simulink model "TST_PIntkVUs_DD"  (R2016b)
settings: Solver=FixedStepDiscrete  StartTime=0.0  StopTime=simTime  FixedStep=sampleTime  RelTol=1e-3
values from neighbouring files (symbols this model uses):
  testCase = 1    [initTST_PIntkVUs_DD_001.m]    (also in initTST_PIntkVUs_DD_002.m = 2; initTST_PIntkVUs_DD_003.m = 3; initTST_PIntkVUs_DD_004.m = 4; initTST_PIntkVUs_DD_005.m = 5)
libraries: UnitTest_Lib x98, simulink x8
(part 3 of 3)

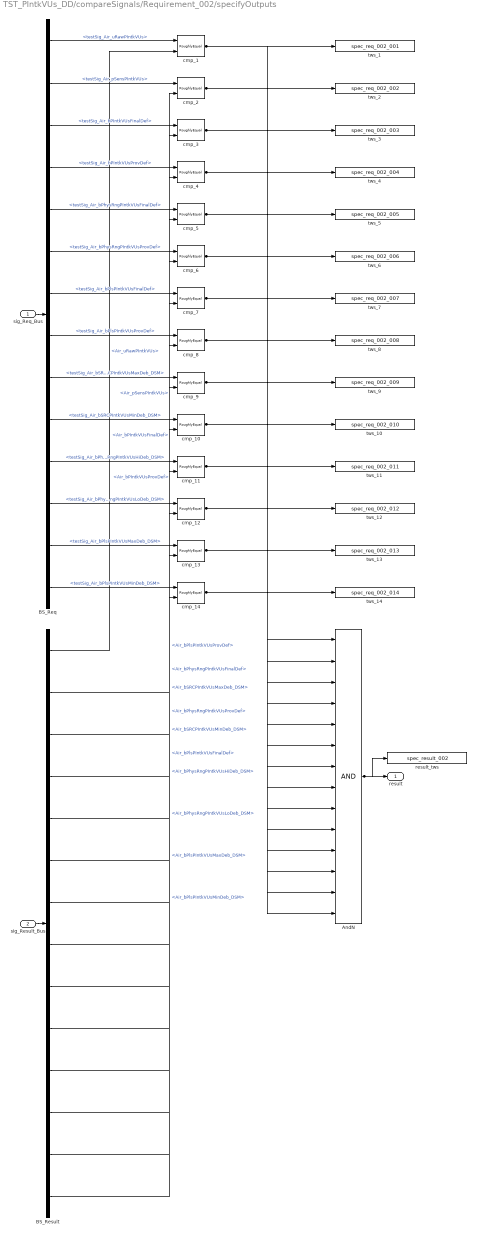
== system TST_PIntkVUs_DD/compareSignals/Requirement_002/specifyOutputs ==
  sig_Req_Bus : Inport
  sig_Result_Bus : Inport  Port=2
  AndN : Logic  Inputs=14
  BS_Req : BusSelector  OutputSignals=testSig_Air_uRawPIntkVUs,testSig_Air_pSensPIntkVUs,testSig_Air_bPIntkVUsFinalDef,testSig_Air_bPIntkVUsProvDef,testSig_Air_bPhysRngPIntkVUsFinalDef,testSig_Air_bPhysRngPIntkVUsProvDef,testSig_Air_bPlsPIntkVUsFinalDef,testSig_Air_bPlsPIntkVUsProvDef,testSig_Air_bSRCPIntkVUsMaxDeb_DSM,testSig_Air_bSRCPIntkVUsMinDeb_DSM,testSig_Air_bPhysRngPIntkVUsHiDeb_DSM,testSig_Air_bPhysRngPIntkVUsLoDeb_DSM,testSig_Air_bPlsPIntkVUsMaxDeb_DSM,testSig_Air_bPlsPIntkVUsMinDeb_DSM
  BS_Result : BusSelector  OutputSignals=Air_uRawPIntkVUs,Air_pSensPIntkVUs,Air_bPIntkVUsFinalDef,Air_bPIntkVUsProvDef,Air_bPhysRngPIntkVUsFinalDef,Air_bPhysRngPIntkVUsProvDef,Air_bPlsPIntkVUsFinalDef,Air_bPlsPIntkVUsProvDef,Air_bSRCPIntkVUsMaxDeb_DSM,Air_bSRCPIntkVUsMinDeb_DSM,Air_bPhysRngPIntkVUsHiDeb_DSM,Air_bPhysRngPIntkVUsLoDeb_DSM,Air_bPlsPIntkVUsMaxDeb_DSM,Air_bPlsPIntkVUsMinDeb_DSM
  cmp_{1..14} (14 alike) : UnitTest_Lib/RoughlyEqual  slope=0.1
  result_tws : ToWorkspace  VariableName=spec_result_002
  tws_1 : ToWorkspace  VariableName=spec_req_002_001
  tws_10 : ToWorkspace  VariableName=spec_req_002_010
  tws_11 : ToWorkspace  VariableName=spec_req_002_011
  tws_12 : ToWorkspace  VariableName=spec_req_002_012
  tws_13 : ToWorkspace  VariableName=spec_req_002_013
  tws_14 : ToWorkspace  VariableName=spec_req_002_014
  tws_2 : ToWorkspace  VariableName=spec_req_002_002
  tws_3 : ToWorkspace  VariableName=spec_req_002_003
  tws_4 : ToWorkspace  VariableName=spec_req_002_004
  tws_5 : ToWorkspace  VariableName=spec_req_002_005
  tws_6 : ToWorkspace  VariableName=spec_req_002_006
  tws_7 : ToWorkspace  VariableName=spec_req_002_007
  tws_8 : ToWorkspace  VariableName=spec_req_002_008
  tws_9 : ToWorkspace  VariableName=spec_req_002_009
  result : Outport
  wires:
  sig_Req_Bus/1 -> BS_Req/1
  sig_Result_Bus/1 -> BS_Result/1
  AndN/1 -> result/1, result_tws/1
  BS_Req/1 -> cmp_1/1  "<testSig_Air_uRawPIntkVUs>"
  BS_Result/1 -> cmp_1/2  "<Air_uRawPIntkVUs>"
  cmp_1/1 -> tws_1/1, AndN/1
  BS_Req/2 -> cmp_2/1  "<testSig_Air_pSensPIntkVUs>"
  BS_Result/2 -> cmp_2/2  "<Air_pSensPIntkVUs>"
  cmp_2/1 -> tws_2/1, AndN/2
  BS_Req/3 -> cmp_3/1  "<testSig_Air_bPIntkVUsFinalDef>"
  BS_Result/3 -> cmp_3/2  "<Air_bPIntkVUsFinalDef>"
  cmp_3/1 -> tws_3/1, AndN/3
  BS_Req/4 -> cmp_4/1  "<testSig_Air_bPIntkVUsProvDef>"
  BS_Result/4 -> cmp_4/2  "<Air_bPIntkVUsProvDef>"
  cmp_4/1 -> tws_4/1, AndN/4
  BS_Req/5 -> cmp_5/1  "<testSig_Air_bPhysRngPIntkVUsFinalDef>"
  BS_Result/5 -> cmp_5/2  "<Air_bPhysRngPIntkVUsFinalDef>"
  cmp_5/1 -> tws_5/1, AndN/5
  BS_Req/6 -> cmp_6/1  "<testSig_Air_bPhysRngPIntkVUsProvDef>"
  BS_Result/6 -> cmp_6/2  "<Air_bPhysRngPIntkVUsProvDef>"
  cmp_6/1 -> tws_6/1, AndN/6
  BS_Req/7 -> cmp_7/1  "<testSig_Air_bPlsPIntkVUsFinalDef>"
  BS_Result/7 -> cmp_7/2  "<Air_bPlsPIntkVUsFinalDef>"
  cmp_7/1 -> tws_7/1, AndN/7
  BS_Req/8 -> cmp_8/1  "<testSig_Air_bPlsPIntkVUsProvDef>"
  BS_Result/8 -> cmp_8/2  "<Air_bPlsPIntkVUsProvDef>"
  cmp_8/1 -> tws_8/1, AndN/8
  BS_Req/9 -> cmp_9/1  "<testSig_Air_bSRCPIntkVUsMaxDeb_DSM>"
  BS_Result/9 -> cmp_9/2  "<Air_bSRCPIntkVUsMaxDeb_DSM>"
  cmp_9/1 -> tws_9/1, AndN/9
  BS_Req/10 -> cmp_10/1  "<testSig_Air_bSRCPIntkVUsMinDeb_DSM>"
  BS_Result/10 -> cmp_10/2  "<Air_bSRCPIntkVUsMinDeb_DSM>"
  cmp_10/1 -> tws_10/1, AndN/10
  BS_Req/11 -> cmp_11/1  "<testSig_Air_bPhysRngPIntkVUsHiDeb_DSM>"
  BS_Result/11 -> cmp_11/2  "<Air_bPhysRngPIntkVUsHiDeb_DSM>"
  cmp_11/1 -> tws_11/1, AndN/11
  BS_Req/12 -> cmp_12/1  "<testSig_Air_bPhysRngPIntkVUsLoDeb_DSM>"
  BS_Result/12 -> cmp_12/2  "<Air_bPhysRngPIntkVUsLoDeb_DSM>"
  cmp_12/1 -> tws_12/1, AndN/12
  BS_Req/13 -> cmp_13/1  "<testSig_Air_bPlsPIntkVUsMaxDeb_DSM>"
  BS_Result/13 -> cmp_13/2  "<Air_bPlsPIntkVUsMaxDeb_DSM>"
  cmp_13/1 -> tws_13/1, AndN/13
  BS_Req/14 -> cmp_14/1  "<testSig_Air_bPlsPIntkVUsMinDeb_DSM>"
  BS_Result/14 -> cmp_14/2  "<Air_bPlsPIntkVUsMinDeb_DSM>"
  cmp_14/1 -> tws_14/1, AndN/14

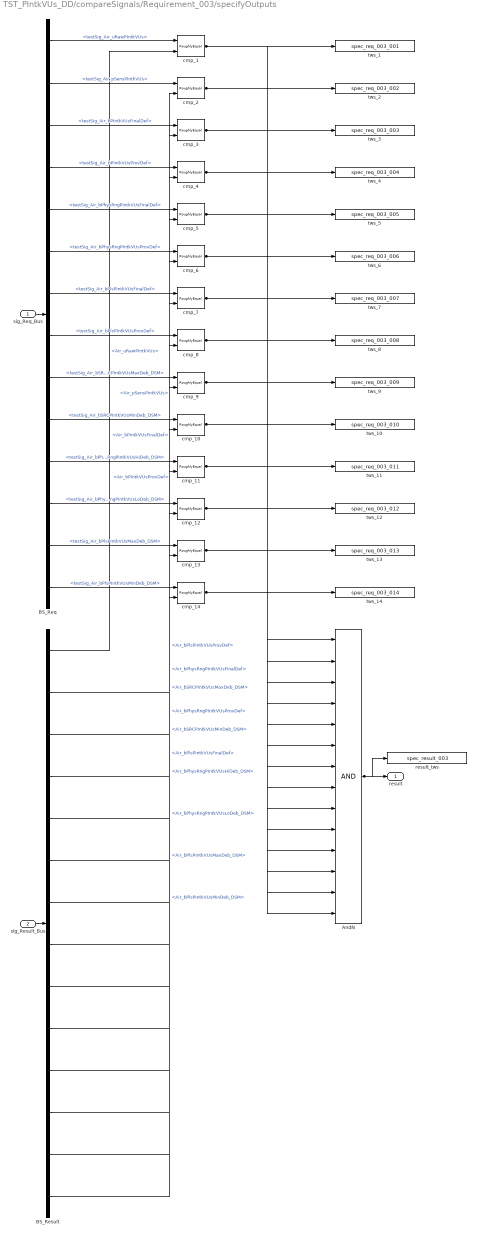
== system TST_PIntkVUs_DD/compareSignals/Requirement_003/specifyOutputs ==
  sig_Req_Bus : Inport
  sig_Result_Bus : Inport  Port=2
  AndN : Logic  Inputs=14
  BS_Req : BusSelector  OutputSignals=testSig_Air_uRawPIntkVUs,testSig_Air_pSensPIntkVUs,testSig_Air_bPIntkVUsFinalDef,testSig_Air_bPIntkVUsProvDef,testSig_Air_bPhysRngPIntkVUsFinalDef,testSig_Air_bPhysRngPIntkVUsProvDef,testSig_Air_bPlsPIntkVUsFinalDef,testSig_Air_bPlsPIntkVUsProvDef,testSig_Air_bSRCPIntkVUsMaxDeb_DSM,testSig_Air_bSRCPIntkVUsMinDeb_DSM,testSig_Air_bPhysRngPIntkVUsHiDeb_DSM,testSig_Air_bPhysRngPIntkVUsLoDeb_DSM,testSig_Air_bPlsPIntkVUsMaxDeb_DSM,testSig_Air_bPlsPIntkVUsMinDeb_DSM
  BS_Result : BusSelector  OutputSignals=Air_uRawPIntkVUs,Air_pSensPIntkVUs,Air_bPIntkVUsFinalDef,Air_bPIntkVUsProvDef,Air_bPhysRngPIntkVUsFinalDef,Air_bPhysRngPIntkVUsProvDef,Air_bPlsPIntkVUsFinalDef,Air_bPlsPIntkVUsProvDef,Air_bSRCPIntkVUsMaxDeb_DSM,Air_bSRCPIntkVUsMinDeb_DSM,Air_bPhysRngPIntkVUsHiDeb_DSM,Air_bPhysRngPIntkVUsLoDeb_DSM,Air_bPlsPIntkVUsMaxDeb_DSM,Air_bPlsPIntkVUsMinDeb_DSM
  cmp_{1..14} (14 alike) : UnitTest_Lib/RoughlyEqual  slope=0.1
  result_tws : ToWorkspace  VariableName=spec_result_003
  tws_1 : ToWorkspace  VariableName=spec_req_003_001
  tws_10 : ToWorkspace  VariableName=spec_req_003_010
  tws_11 : ToWorkspace  VariableName=spec_req_003_011
  tws_12 : ToWorkspace  VariableName=spec_req_003_012
  tws_13 : ToWorkspace  VariableName=spec_req_003_013
  tws_14 : ToWorkspace  VariableName=spec_req_003_014
  tws_2 : ToWorkspace  VariableName=spec_req_003_002
  tws_3 : ToWorkspace  VariableName=spec_req_003_003
  tws_4 : ToWorkspace  VariableName=spec_req_003_004
  tws_5 : ToWorkspace  VariableName=spec_req_003_005
  tws_6 : ToWorkspace  VariableName=spec_req_003_006
  tws_7 : ToWorkspace  VariableName=spec_req_003_007
  tws_8 : ToWorkspace  VariableName=spec_req_003_008
  tws_9 : ToWorkspace  VariableName=spec_req_003_009
  result : Outport
  wires:
  sig_Req_Bus/1 -> BS_Req/1
  sig_Result_Bus/1 -> BS_Result/1
  AndN/1 -> result/1, result_tws/1
  BS_Req/1 -> cmp_1/1  "<testSig_Air_uRawPIntkVUs>"
  BS_Result/1 -> cmp_1/2  "<Air_uRawPIntkVUs>"
  cmp_1/1 -> tws_1/1, AndN/1
  BS_Req/2 -> cmp_2/1  "<testSig_Air_pSensPIntkVUs>"
  BS_Result/2 -> cmp_2/2  "<Air_pSensPIntkVUs>"
  cmp_2/1 -> tws_2/1, AndN/2
  BS_Req/3 -> cmp_3/1  "<testSig_Air_bPIntkVUsFinalDef>"
  BS_Result/3 -> cmp_3/2  "<Air_bPIntkVUsFinalDef>"
  cmp_3/1 -> tws_3/1, AndN/3
  BS_Req/4 -> cmp_4/1  "<testSig_Air_bPIntkVUsProvDef>"
  BS_Result/4 -> cmp_4/2  "<Air_bPIntkVUsProvDef>"
  cmp_4/1 -> tws_4/1, AndN/4
  BS_Req/5 -> cmp_5/1  "<testSig_Air_bPhysRngPIntkVUsFinalDef>"
  BS_Result/5 -> cmp_5/2  "<Air_bPhysRngPIntkVUsFinalDef>"
  cmp_5/1 -> tws_5/1, AndN/5
  BS_Req/6 -> cmp_6/1  "<testSig_Air_bPhysRngPIntkVUsProvDef>"
  BS_Result/6 -> cmp_6/2  "<Air_bPhysRngPIntkVUsProvDef>"
  cmp_6/1 -> tws_6/1, AndN/6
  BS_Req/7 -> cmp_7/1  "<testSig_Air_bPlsPIntkVUsFinalDef>"
  BS_Result/7 -> cmp_7/2  "<Air_bPlsPIntkVUsFinalDef>"
  cmp_7/1 -> tws_7/1, AndN/7
  BS_Req/8 -> cmp_8/1  "<testSig_Air_bPlsPIntkVUsProvDef>"
  BS_Result/8 -> cmp_8/2  "<Air_bPlsPIntkVUsProvDef>"
  cmp_8/1 -> tws_8/1, AndN/8
  BS_Req/9 -> cmp_9/1  "<testSig_Air_bSRCPIntkVUsMaxDeb_DSM>"
  BS_Result/9 -> cmp_9/2  "<Air_bSRCPIntkVUsMaxDeb_DSM>"
  cmp_9/1 -> tws_9/1, AndN/9
  BS_Req/10 -> cmp_10/1  "<testSig_Air_bSRCPIntkVUsMinDeb_DSM>"
  BS_Result/10 -> cmp_10/2  "<Air_bSRCPIntkVUsMinDeb_DSM>"
  cmp_10/1 -> tws_10/1, AndN/10
  BS_Req/11 -> cmp_11/1  "<testSig_Air_bPhysRngPIntkVUsHiDeb_DSM>"
  BS_Result/11 -> cmp_11/2  "<Air_bPhysRngPIntkVUsHiDeb_DSM>"
  cmp_11/1 -> tws_11/1, AndN/11
  BS_Req/12 -> cmp_12/1  "<testSig_Air_bPhysRngPIntkVUsLoDeb_DSM>"
  BS_Result/12 -> cmp_12/2  "<Air_bPhysRngPIntkVUsLoDeb_DSM>"
  cmp_12/1 -> tws_12/1, AndN/12
  BS_Req/13 -> cmp_13/1  "<testSig_Air_bPlsPIntkVUsMaxDeb_DSM>"
  BS_Result/13 -> cmp_13/2  "<Air_bPlsPIntkVUsMaxDeb_DSM>"
  cmp_13/1 -> tws_13/1, AndN/13
  BS_Req/14 -> cmp_14/1  "<testSig_Air_bPlsPIntkVUsMinDeb_DSM>"
  BS_Result/14 -> cmp_14/2  "<Air_bPlsPIntkVUsMinDeb_DSM>"
  cmp_14/1 -> tws_14/1, AndN/14

== system TST_PIntkVUs_DD/compareSignals/Requirement_004/specifyOutputs ==
  sig_Req_Bus : Inport
  sig_Result_Bus : Inport  Port=2
  AndN : Logic  Inputs=14
  BS_Req : BusSelector  OutputSignals=testSig_Air_uRawPIntkVUs,testSig_Air_pSensPIntkVUs,testSig_Air_bPIntkVUsFinalDef,testSig_Air_bPIntkVUsProvDef,testSig_Air_bPhysRngPIntkVUsFinalDef,testSig_Air_bPhysRngPIntkVUsProvDef,testSig_Air_bPlsPIntkVUsFinalDef,testSig_Air_bPlsPIntkVUsProvDef,testSig_Air_bSRCPIntkVUsMaxDeb_DSM,testSig_Air_bSRCPIntkVUsMinDeb_DSM,testSig_Air_bPhysRngPIntkVUsHiDeb_DSM,testSig_Air_bPhysRngPIntkVUsLoDeb_DSM,testSig_Air_bPlsPIntkVUsMaxDeb_DSM,testSig_Air_bPlsPIntkVUsMinDeb_DSM
  BS_Result : BusSelector  OutputSignals=Air_uRawPIntkVUs,Air_pSensPIntkVUs,Air_bPIntkVUsFinalDef,Air_bPIntkVUsProvDef,Air_bPhysRngPIntkVUsFinalDef,Air_bPhysRngPIntkVUsProvDef,Air_bPlsPIntkVUsFinalDef,Air_bPlsPIntkVUsProvDef,Air_bSRCPIntkVUsMaxDeb_DSM,Air_bSRCPIntkVUsMinDeb_DSM,Air_bPhysRngPIntkVUsHiDeb_DSM,Air_bPhysRngPIntkVUsLoDeb_DSM,Air_bPlsPIntkVUsMaxDeb_DSM,Air_bPlsPIntkVUsMinDeb_DSM
  cmp_{1..14} (14 alike) : UnitTest_Lib/RoughlyEqual  slope=0.1
  result_tws : ToWorkspace  VariableName=spec_result_004
  tws_1 : ToWorkspace  VariableName=spec_req_004_001
  tws_10 : ToWorkspace  VariableName=spec_req_004_010
  tws_11 : ToWorkspace  VariableName=spec_req_004_011
  tws_12 : ToWorkspace  VariableName=spec_req_004_012
  tws_13 : ToWorkspace  VariableName=spec_req_004_013
  tws_14 : ToWorkspace  VariableName=spec_req_004_014
  tws_2 : ToWorkspace  VariableName=spec_req_004_002
  tws_3 : ToWorkspace  VariableName=spec_req_004_003
  tws_4 : ToWorkspace  VariableName=spec_req_004_004
  tws_5 : ToWorkspace  VariableName=spec_req_004_005
  tws_6 : ToWorkspace  VariableName=spec_req_004_006
  tws_7 : ToWorkspace  VariableName=spec_req_004_007
  tws_8 : ToWorkspace  VariableName=spec_req_004_008
  tws_9 : ToWorkspace  VariableName=spec_req_004_009
  result : Outport
  wires:
  sig_Req_Bus/1 -> BS_Req/1
  sig_Result_Bus/1 -> BS_Result/1
  AndN/1 -> result/1, result_tws/1
  BS_Req/1 -> cmp_1/1  "<testSig_Air_uRawPIntkVUs>"
  BS_Result/1 -> cmp_1/2  "<Air_uRawPIntkVUs>"
  cmp_1/1 -> tws_1/1, AndN/1
  BS_Req/2 -> cmp_2/1  "<testSig_Air_pSensPIntkVUs>"
  BS_Result/2 -> cmp_2/2  "<Air_pSensPIntkVUs>"
  cmp_2/1 -> tws_2/1, AndN/2
  BS_Req/3 -> cmp_3/1  "<testSig_Air_bPIntkVUsFinalDef>"
  BS_Result/3 -> cmp_3/2  "<Air_bPIntkVUsFinalDef>"
  cmp_3/1 -> tws_3/1, AndN/3
  BS_Req/4 -> cmp_4/1  "<testSig_Air_bPIntkVUsProvDef>"
  BS_Result/4 -> cmp_4/2  "<Air_bPIntkVUsProvDef>"
  cmp_4/1 -> tws_4/1, AndN/4
  BS_Req/5 -> cmp_5/1  "<testSig_Air_bPhysRngPIntkVUsFinalDef>"
  BS_Result/5 -> cmp_5/2  "<Air_bPhysRngPIntkVUsFinalDef>"
  cmp_5/1 -> tws_5/1, AndN/5
  BS_Req/6 -> cmp_6/1  "<testSig_Air_bPhysRngPIntkVUsProvDef>"
  BS_Result/6 -> cmp_6/2  "<Air_bPhysRngPIntkVUsProvDef>"
  cmp_6/1 -> tws_6/1, AndN/6
  BS_Req/7 -> cmp_7/1  "<testSig_Air_bPlsPIntkVUsFinalDef>"
  BS_Result/7 -> cmp_7/2  "<Air_bPlsPIntkVUsFinalDef>"
  cmp_7/1 -> tws_7/1, AndN/7
  BS_Req/8 -> cmp_8/1  "<testSig_Air_bPlsPIntkVUsProvDef>"
  BS_Result/8 -> cmp_8/2  "<Air_bPlsPIntkVUsProvDef>"
  cmp_8/1 -> tws_8/1, AndN/8
  BS_Req/9 -> cmp_9/1  "<testSig_Air_bSRCPIntkVUsMaxDeb_DSM>"
  BS_Result/9 -> cmp_9/2  "<Air_bSRCPIntkVUsMaxDeb_DSM>"
  cmp_9/1 -> tws_9/1, AndN/9
  BS_Req/10 -> cmp_10/1  "<testSig_Air_bSRCPIntkVUsMinDeb_DSM>"
  BS_Result/10 -> cmp_10/2  "<Air_bSRCPIntkVUsMinDeb_DSM>"
  cmp_10/1 -> tws_10/1, AndN/10
  BS_Req/11 -> cmp_11/1  "<testSig_Air_bPhysRngPIntkVUsHiDeb_DSM>"
  BS_Result/11 -> cmp_11/2  "<Air_bPhysRngPIntkVUsHiDeb_DSM>"
  cmp_11/1 -> tws_11/1, AndN/11
  BS_Req/12 -> cmp_12/1  "<testSig_Air_bPhysRngPIntkVUsLoDeb_DSM>"
  BS_Result/12 -> cmp_12/2  "<Air_bPhysRngPIntkVUsLoDeb_DSM>"
  cmp_12/1 -> tws_12/1, AndN/12
  BS_Req/13 -> cmp_13/1  "<testSig_Air_bPlsPIntkVUsMaxDeb_DSM>"
  BS_Result/13 -> cmp_13/2  "<Air_bPlsPIntkVUsMaxDeb_DSM>"
  cmp_13/1 -> tws_13/1, AndN/13
  BS_Req/14 -> cmp_14/1  "<testSig_Air_bPlsPIntkVUsMinDeb_DSM>"
  BS_Result/14 -> cmp_14/2  "<Air_bPlsPIntkVUsMinDeb_DSM>"
  cmp_14/1 -> tws_14/1, AndN/14

== system TST_PIntkVUs_DD/compareSignals/Requirement_005/specifyOutputs ==
  sig_Req_Bus : Inport
  sig_Result_Bus : Inport  Port=2
  AndN : Logic  Inputs=14
  BS_Req : BusSelector  OutputSignals=testSig_Air_uRawPIntkVUs,testSig_Air_pSensPIntkVUs,testSig_Air_bPIntkVUsFinalDef,testSig_Air_bPIntkVUsProvDef,testSig_Air_bPhysRngPIntkVUsFinalDef,testSig_Air_bPhysRngPIntkVUsProvDef,testSig_Air_bPlsPIntkVUsFinalDef,testSig_Air_bPlsPIntkVUsProvDef,testSig_Air_bSRCPIntkVUsMaxDeb_DSM,testSig_Air_bSRCPIntkVUsMinDeb_DSM,testSig_Air_bPhysRngPIntkVUsHiDeb_DSM,testSig_Air_bPhysRngPIntkVUsLoDeb_DSM,testSig_Air_bPlsPIntkVUsMaxDeb_DSM,testSig_Air_bPlsPIntkVUsMinDeb_DSM
  BS_Result : BusSelector  OutputSignals=Air_uRawPIntkVUs,Air_pSensPIntkVUs,Air_bPIntkVUsFinalDef,Air_bPIntkVUsProvDef,Air_bPhysRngPIntkVUsFinalDef,Air_bPhysRngPIntkVUsProvDef,Air_bPlsPIntkVUsFinalDef,Air_bPlsPIntkVUsProvDef,Air_bSRCPIntkVUsMaxDeb_DSM,Air_bSRCPIntkVUsMinDeb_DSM,Air_bPhysRngPIntkVUsHiDeb_DSM,Air_bPhysRngPIntkVUsLoDeb_DSM,Air_bPlsPIntkVUsMaxDeb_DSM,Air_bPlsPIntkVUsMinDeb_DSM
  cmp_{1..14} (14 alike) : UnitTest_Lib/RoughlyEqual  slope=0.1
  result_tws : ToWorkspace  VariableName=spec_result_005
  tws_1 : ToWorkspace  VariableName=spec_req_005_001
  tws_10 : ToWorkspace  VariableName=spec_req_005_010
  tws_11 : ToWorkspace  VariableName=spec_req_005_011
  tws_12 : ToWorkspace  VariableName=spec_req_005_012
  tws_13 : ToWorkspace  VariableName=spec_req_005_013
  tws_14 : ToWorkspace  VariableName=spec_req_005_014
  tws_2 : ToWorkspace  VariableName=spec_req_005_002
  tws_3 : ToWorkspace  VariableName=spec_req_005_003
  tws_4 : ToWorkspace  VariableName=spec_req_005_004
  tws_5 : ToWorkspace  VariableName=spec_req_005_005
  tws_6 : ToWorkspace  VariableName=spec_req_005_006
  tws_7 : ToWorkspace  VariableName=spec_req_005_007
  tws_8 : ToWorkspace  VariableName=spec_req_005_008
  tws_9 : ToWorkspace  VariableName=spec_req_005_009
  result : Outport
  wires:
  sig_Req_Bus/1 -> BS_Req/1
  sig_Result_Bus/1 -> BS_Result/1
  AndN/1 -> result/1, result_tws/1
  BS_Req/1 -> cmp_1/1  "<testSig_Air_uRawPIntkVUs>"
  BS_Result/1 -> cmp_1/2  "<Air_uRawPIntkVUs>"
  cmp_1/1 -> tws_1/1, AndN/1
  BS_Req/2 -> cmp_2/1  "<testSig_Air_pSensPIntkVUs>"
  BS_Result/2 -> cmp_2/2  "<Air_pSensPIntkVUs>"
  cmp_2/1 -> tws_2/1, AndN/2
  BS_Req/3 -> cmp_3/1  "<testSig_Air_bPIntkVUsFinalDef>"
  BS_Result/3 -> cmp_3/2  "<Air_bPIntkVUsFinalDef>"
  cmp_3/1 -> tws_3/1, AndN/3
  BS_Req/4 -> cmp_4/1  "<testSig_Air_bPIntkVUsProvDef>"
  BS_Result/4 -> cmp_4/2  "<Air_bPIntkVUsProvDef>"
  cmp_4/1 -> tws_4/1, AndN/4
  BS_Req/5 -> cmp_5/1  "<testSig_Air_bPhysRngPIntkVUsFinalDef>"
  BS_Result/5 -> cmp_5/2  "<Air_bPhysRngPIntkVUsFinalDef>"
  cmp_5/1 -> tws_5/1, AndN/5
  BS_Req/6 -> cmp_6/1  "<testSig_Air_bPhysRngPIntkVUsProvDef>"
  BS_Result/6 -> cmp_6/2  "<Air_bPhysRngPIntkVUsProvDef>"
  cmp_6/1 -> tws_6/1, AndN/6
  BS_Req/7 -> cmp_7/1  "<testSig_Air_bPlsPIntkVUsFinalDef>"
  BS_Result/7 -> cmp_7/2  "<Air_bPlsPIntkVUsFinalDef>"
  cmp_7/1 -> tws_7/1, AndN/7
  BS_Req/8 -> cmp_8/1  "<testSig_Air_bPlsPIntkVUsProvDef>"
  BS_Result/8 -> cmp_8/2  "<Air_bPlsPIntkVUsProvDef>"
  cmp_8/1 -> tws_8/1, AndN/8
  BS_Req/9 -> cmp_9/1  "<testSig_Air_bSRCPIntkVUsMaxDeb_DSM>"
  BS_Result/9 -> cmp_9/2  "<Air_bSRCPIntkVUsMaxDeb_DSM>"
  cmp_9/1 -> tws_9/1, AndN/9
  BS_Req/10 -> cmp_10/1  "<testSig_Air_bSRCPIntkVUsMinDeb_DSM>"
  BS_Result/10 -> cmp_10/2  "<Air_bSRCPIntkVUsMinDeb_DSM>"
  cmp_10/1 -> tws_10/1, AndN/10
  BS_Req/11 -> cmp_11/1  "<testSig_Air_bPhysRngPIntkVUsHiDeb_DSM>"
  BS_Result/11 -> cmp_11/2  "<Air_bPhysRngPIntkVUsHiDeb_DSM>"
  cmp_11/1 -> tws_11/1, AndN/11
  BS_Req/12 -> cmp_12/1  "<testSig_Air_bPhysRngPIntkVUsLoDeb_DSM>"
  BS_Result/12 -> cmp_12/2  "<Air_bPhysRngPIntkVUsLoDeb_DSM>"
  cmp_12/1 -> tws_12/1, AndN/12
  BS_Req/13 -> cmp_13/1  "<testSig_Air_bPlsPIntkVUsMaxDeb_DSM>"
  BS_Result/13 -> cmp_13/2  "<Air_bPlsPIntkVUsMaxDeb_DSM>"
  cmp_13/1 -> tws_13/1, AndN/13
  BS_Req/14 -> cmp_14/1  "<testSig_Air_bPlsPIntkVUsMinDeb_DSM>"
  BS_Result/14 -> cmp_14/2  "<Air_bPlsPIntkVUsMinDeb_DSM>"
  cmp_14/1 -> tws_14/1, AndN/14

== system TST_PIntkVUs_DD/compareSignals/Requirement_006/specifyOutputs ==
  sig_Req_Bus : Inport
  sig_Result_Bus : Inport  Port=2
  AndN : Logic  Inputs=14
  BS_Req : BusSelector  OutputSignals=testSig_Air_uRawPIntkVUs,testSig_Air_pSensPIntkVUs,testSig_Air_bPIntkVUsFinalDef,testSig_Air_bPIntkVUsProvDef,testSig_Air_bPhysRngPIntkVUsFinalDef,testSig_Air_bPhysRngPIntkVUsProvDef,testSig_Air_bPlsPIntkVUsFinalDef,testSig_Air_bPlsPIntkVUsProvDef,testSig_Air_bSRCPIntkVUsMaxDeb_DSM,testSig_Air_bSRCPIntkVUsMinDeb_DSM,testSig_Air_bPhysRngPIntkVUsHiDeb_DSM,testSig_Air_bPhysRngPIntkVUsLoDeb_DSM,testSig_Air_bPlsPIntkVUsMaxDeb_DSM,testSig_Air_bPlsPIntkVUsMinDeb_DSM
  BS_Result : BusSelector  OutputSignals=Air_uRawPIntkVUs,Air_pSensPIntkVUs,Air_bPIntkVUsFinalDef,Air_bPIntkVUsProvDef,Air_bPhysRngPIntkVUsFinalDef,Air_bPhysRngPIntkVUsProvDef,Air_bPlsPIntkVUsFinalDef,Air_bPlsPIntkVUsProvDef,Air_bSRCPIntkVUsMaxDeb_DSM,Air_bSRCPIntkVUsMinDeb_DSM,Air_bPhysRngPIntkVUsHiDeb_DSM,Air_bPhysRngPIntkVUsLoDeb_DSM,Air_bPlsPIntkVUsMaxDeb_DSM,Air_bPlsPIntkVUsMinDeb_DSM
  cmp_{1..14} (14 alike) : UnitTest_Lib/RoughlyEqual  slope=0.1
  result_tws : ToWorkspace  VariableName=spec_result_006
  tws_1 : ToWorkspace  VariableName=spec_req_006_001
  tws_10 : ToWorkspace  VariableName=spec_req_006_010
  tws_11 : ToWorkspace  VariableName=spec_req_006_011
  tws_12 : ToWorkspace  VariableName=spec_req_006_012
  tws_13 : ToWorkspace  VariableName=spec_req_006_013
  tws_14 : ToWorkspace  VariableName=spec_req_006_014
  tws_2 : ToWorkspace  VariableName=spec_req_006_002
  tws_3 : ToWorkspace  VariableName=spec_req_006_003
  tws_4 : ToWorkspace  VariableName=spec_req_006_004
  tws_5 : ToWorkspace  VariableName=spec_req_006_005
  tws_6 : ToWorkspace  VariableName=spec_req_006_006
  tws_7 : ToWorkspace  VariableName=spec_req_006_007
  tws_8 : ToWorkspace  VariableName=spec_req_006_008
  tws_9 : ToWorkspace  VariableName=spec_req_006_009
  result : Outport
  wires:
  sig_Req_Bus/1 -> BS_Req/1
  sig_Result_Bus/1 -> BS_Result/1
  AndN/1 -> result/1, result_tws/1
  BS_Req/1 -> cmp_1/1  "<testSig_Air_uRawPIntkVUs>"
  BS_Result/1 -> cmp_1/2  "<Air_uRawPIntkVUs>"
  cmp_1/1 -> tws_1/1, AndN/1
  BS_Req/2 -> cmp_2/1  "<testSig_Air_pSensPIntkVUs>"
  BS_Result/2 -> cmp_2/2  "<Air_pSensPIntkVUs>"
  cmp_2/1 -> tws_2/1, AndN/2
  BS_Req/3 -> cmp_3/1  "<testSig_Air_bPIntkVUsFinalDef>"
  BS_Result/3 -> cmp_3/2  "<Air_bPIntkVUsFinalDef>"
  cmp_3/1 -> tws_3/1, AndN/3
  BS_Req/4 -> cmp_4/1  "<testSig_Air_bPIntkVUsProvDef>"
  BS_Result/4 -> cmp_4/2  "<Air_bPIntkVUsProvDef>"
  cmp_4/1 -> tws_4/1, AndN/4
  BS_Req/5 -> cmp_5/1  "<testSig_Air_bPhysRngPIntkVUsFinalDef>"
  BS_Result/5 -> cmp_5/2  "<Air_bPhysRngPIntkVUsFinalDef>"
  cmp_5/1 -> tws_5/1, AndN/5
  BS_Req/6 -> cmp_6/1  "<testSig_Air_bPhysRngPIntkVUsProvDef>"
  BS_Result/6 -> cmp_6/2  "<Air_bPhysRngPIntkVUsProvDef>"
  cmp_6/1 -> tws_6/1, AndN/6
  BS_Req/7 -> cmp_7/1  "<testSig_Air_bPlsPIntkVUsFinalDef>"
  BS_Result/7 -> cmp_7/2  "<Air_bPlsPIntkVUsFinalDef>"
  cmp_7/1 -> tws_7/1, AndN/7
  BS_Req/8 -> cmp_8/1  "<testSig_Air_bPlsPIntkVUsProvDef>"
  BS_Result/8 -> cmp_8/2  "<Air_bPlsPIntkVUsProvDef>"
  cmp_8/1 -> tws_8/1, AndN/8
  BS_Req/9 -> cmp_9/1  "<testSig_Air_bSRCPIntkVUsMaxDeb_DSM>"
  BS_Result/9 -> cmp_9/2  "<Air_bSRCPIntkVUsMaxDeb_DSM>"
  cmp_9/1 -> tws_9/1, AndN/9
  BS_Req/10 -> cmp_10/1  "<testSig_Air_bSRCPIntkVUsMinDeb_DSM>"
  BS_Result/10 -> cmp_10/2  "<Air_bSRCPIntkVUsMinDeb_DSM>"
  cmp_10/1 -> tws_10/1, AndN/10
  BS_Req/11 -> cmp_11/1  "<testSig_Air_bPhysRngPIntkVUsHiDeb_DSM>"
  BS_Result/11 -> cmp_11/2  "<Air_bPhysRngPIntkVUsHiDeb_DSM>"
  cmp_11/1 -> tws_11/1, AndN/11
  BS_Req/12 -> cmp_12/1  "<testSig_Air_bPhysRngPIntkVUsLoDeb_DSM>"
  BS_Result/12 -> cmp_12/2  "<Air_bPhysRngPIntkVUsLoDeb_DSM>"
  cmp_12/1 -> tws_12/1, AndN/12
  BS_Req/13 -> cmp_13/1  "<testSig_Air_bPlsPIntkVUsMaxDeb_DSM>"
  BS_Result/13 -> cmp_13/2  "<Air_bPlsPIntkVUsMaxDeb_DSM>"
  cmp_13/1 -> tws_13/1, AndN/13
  BS_Req/14 -> cmp_14/1  "<testSig_Air_bPlsPIntkVUsMinDeb_DSM>"
  BS_Result/14 -> cmp_14/2  "<Air_bPlsPIntkVUsMinDeb_DSM>"
  cmp_14/1 -> tws_14/1, AndN/14

== system TST_PIntkVUs_DD/compareSignals/Requirement_007/specifyOutputs ==
  sig_Req_Bus : Inport
  sig_Result_Bus : Inport  Port=2
  AndN : Logic  Inputs=14
  BS_Req : BusSelector  OutputSignals=testSig_Air_uRawPIntkVUs,testSig_Air_pSensPIntkVUs,testSig_Air_bPIntkVUsFinalDef,testSig_Air_bPIntkVUsProvDef,testSig_Air_bPhysRngPIntkVUsFinalDef,testSig_Air_bPhysRngPIntkVUsProvDef,testSig_Air_bPlsPIntkVUsFinalDef,testSig_Air_bPlsPIntkVUsProvDef,testSig_Air_bSRCPIntkVUsMaxDeb_DSM,testSig_Air_bSRCPIntkVUsMinDeb_DSM,testSig_Air_bPhysRngPIntkVUsHiDeb_DSM,testSig_Air_bPhysRngPIntkVUsLoDeb_DSM,testSig_Air_bPlsPIntkVUsMaxDeb_DSM,testSig_Air_bPlsPIntkVUsMinDeb_DSM
  BS_Result : BusSelector  OutputSignals=Air_uRawPIntkVUs,Air_pSensPIntkVUs,Air_bPIntkVUsFinalDef,Air_bPIntkVUsProvDef,Air_bPhysRngPIntkVUsFinalDef,Air_bPhysRngPIntkVUsProvDef,Air_bPlsPIntkVUsFinalDef,Air_bPlsPIntkVUsProvDef,Air_bSRCPIntkVUsMaxDeb_DSM,Air_bSRCPIntkVUsMinDeb_DSM,Air_bPhysRngPIntkVUsHiDeb_DSM,Air_bPhysRngPIntkVUsLoDeb_DSM,Air_bPlsPIntkVUsMaxDeb_DSM,Air_bPlsPIntkVUsMinDeb_DSM
  cmp_{1..14} (14 alike) : UnitTest_Lib/RoughlyEqual  slope=0.1
  result_tws : ToWorkspace  VariableName=spec_result_007
  tws_1 : ToWorkspace  VariableName=spec_req_007_001
  tws_10 : ToWorkspace  VariableName=spec_req_007_010
  tws_11 : ToWorkspace  VariableName=spec_req_007_011
  tws_12 : ToWorkspace  VariableName=spec_req_007_012
  tws_13 : ToWorkspace  VariableName=spec_req_007_013
  tws_14 : ToWorkspace  VariableName=spec_req_007_014
  tws_2 : ToWorkspace  VariableName=spec_req_007_002
  tws_3 : ToWorkspace  VariableName=spec_req_007_003
  tws_4 : ToWorkspace  VariableName=spec_req_007_004
  tws_5 : ToWorkspace  VariableName=spec_req_007_005
  tws_6 : ToWorkspace  VariableName=spec_req_007_006
  tws_7 : ToWorkspace  VariableName=spec_req_007_007
  tws_8 : ToWorkspace  VariableName=spec_req_007_008
  tws_9 : ToWorkspace  VariableName=spec_req_007_009
  result : Outport
  wires:
  sig_Req_Bus/1 -> BS_Req/1
  sig_Result_Bus/1 -> BS_Result/1
  AndN/1 -> result/1, result_tws/1
  BS_Req/1 -> cmp_1/1  "<testSig_Air_uRawPIntkVUs>"
  BS_Result/1 -> cmp_1/2  "<Air_uRawPIntkVUs>"
  cmp_1/1 -> tws_1/1, AndN/1
  BS_Req/2 -> cmp_2/1  "<testSig_Air_pSensPIntkVUs>"
  BS_Result/2 -> cmp_2/2  "<Air_pSensPIntkVUs>"
  cmp_2/1 -> tws_2/1, AndN/2
  BS_Req/3 -> cmp_3/1  "<testSig_Air_bPIntkVUsFinalDef>"
  BS_Result/3 -> cmp_3/2  "<Air_bPIntkVUsFinalDef>"
  cmp_3/1 -> tws_3/1, AndN/3
  BS_Req/4 -> cmp_4/1  "<testSig_Air_bPIntkVUsProvDef>"
  BS_Result/4 -> cmp_4/2  "<Air_bPIntkVUsProvDef>"
  cmp_4/1 -> tws_4/1, AndN/4
  BS_Req/5 -> cmp_5/1  "<testSig_Air_bPhysRngPIntkVUsFinalDef>"
  BS_Result/5 -> cmp_5/2  "<Air_bPhysRngPIntkVUsFinalDef>"
  cmp_5/1 -> tws_5/1, AndN/5
  BS_Req/6 -> cmp_6/1  "<testSig_Air_bPhysRngPIntkVUsProvDef>"
  BS_Result/6 -> cmp_6/2  "<Air_bPhysRngPIntkVUsProvDef>"
  cmp_6/1 -> tws_6/1, AndN/6
  BS_Req/7 -> cmp_7/1  "<testSig_Air_bPlsPIntkVUsFinalDef>"
  BS_Result/7 -> cmp_7/2  "<Air_bPlsPIntkVUsFinalDef>"
  cmp_7/1 -> tws_7/1, AndN/7
  BS_Req/8 -> cmp_8/1  "<testSig_Air_bPlsPIntkVUsProvDef>"
  BS_Result/8 -> cmp_8/2  "<Air_bPlsPIntkVUsProvDef>"
  cmp_8/1 -> tws_8/1, AndN/8
  BS_Req/9 -> cmp_9/1  "<testSig_Air_bSRCPIntkVUsMaxDeb_DSM>"
  BS_Result/9 -> cmp_9/2  "<Air_bSRCPIntkVUsMaxDeb_DSM>"
  cmp_9/1 -> tws_9/1, AndN/9
  BS_Req/10 -> cmp_10/1  "<testSig_Air_bSRCPIntkVUsMinDeb_DSM>"
  BS_Result/10 -> cmp_10/2  "<Air_bSRCPIntkVUsMinDeb_DSM>"
  cmp_10/1 -> tws_10/1, AndN/10
  BS_Req/11 -> cmp_11/1  "<testSig_Air_bPhysRngPIntkVUsHiDeb_DSM>"
  BS_Result/11 -> cmp_11/2  "<Air_bPhysRngPIntkVUsHiDeb_DSM>"
  cmp_11/1 -> tws_11/1, AndN/11
  BS_Req/12 -> cmp_12/1  "<testSig_Air_bPhysRngPIntkVUsLoDeb_DSM>"
  BS_Result/12 -> cmp_12/2  "<Air_bPhysRngPIntkVUsLoDeb_DSM>"
  cmp_12/1 -> tws_12/1, AndN/12
  BS_Req/13 -> cmp_13/1  "<testSig_Air_bPlsPIntkVUsMaxDeb_DSM>"
  BS_Result/13 -> cmp_13/2  "<Air_bPlsPIntkVUsMaxDeb_DSM>"
  cmp_13/1 -> tws_13/1, AndN/13
  BS_Req/14 -> cmp_14/1  "<testSig_Air_bPlsPIntkVUsMinDeb_DSM>"
  BS_Result/14 -> cmp_14/2  "<Air_bPlsPIntkVUsMinDeb_DSM>"
  cmp_14/1 -> tws_14/1, AndN/14
